simulink model "SLCI1_TP_Ericc3_Modele_Matlab_corrige_LMM"  (R2016b)
settings: Solver=ode3  StartTime=0.0  StopTime=5  FixedStep=0.01  RelTol=1e-3  EnableMultiTasking=on
settings Model: Creator=Mathieu  LastModifiedBy=emiliendurif
settings DataIOCC: LimitDataPoints=on  SaveFormat=Array
settings OptimizationCC: LifeSpan=inf
settings DebuggingCC: SFUnexpectedBacktrackingDiag=warning  SFNoUnconditionalDefaultTransitionDiag=warning  SFExecutionAtInitializationDiag=none
settings HardwareCC: ProdBitPerPointer=32  ProdBitPerSizeT=32  ProdBitPerPtrDiffT=32  ProdLargestAtomicFloat=None  ProdIntDivRoundTo=Undefined  ProdEndianess=Unspecified  ProdWordSize=32  ProdHWDeviceType=32-bit Generic
settings ModelReferenceCC: PropagateSignalLabelsOutOfModel=off
settings GRTTargetCC: TargetLangStandard=C89/C90 (ANSI)  GeneratePreprocessorConditionals=Disable all
settings ConfigComp: CovMetricSettings=dw  CovHtmlReporting=on  CovSaveCumulativeToWorkspaceVar=on  CovSaveSingleToWorkspaceVar=on  CovExternalEMLEnable=off

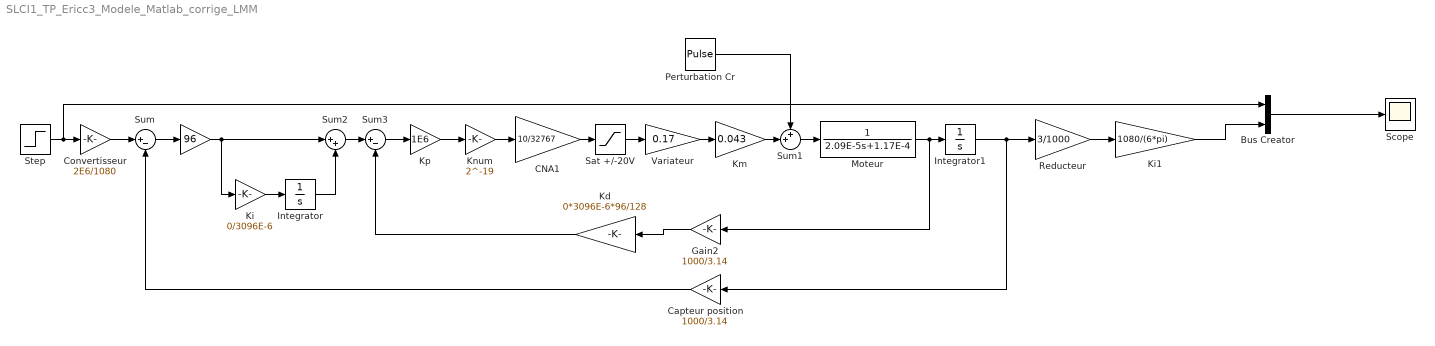
== system SLCI1_TP_Ericc3_Modele_Matlab_corrige_LMM ==
  " " : Gain  Gain=96
  Bus Creator : BusCreator  Inputs=2
  CNA1 : Gain  Gain=10/32767
  "Capteur position " : Gain  Gain=1000/3.14
  Convertisseur : Gain  Gain=2E6/1080
  Gain2 : Gain  Gain=1000/3.14
  Integrator : Integrator
  Integrator1 : Integrator
  Kd : Gain  Gain=0*3096E-6*96/128
  Ki : Gain  Gain=0/3096E-6
  Ki1 : Gain  Gain=1080/(6*pi)
  Km : Gain  Gain=0.043
  Knum : Gain  Gain=2^-19
  Kp : Gain  Gain=1E6
  Moteur : TransferFcn  Denominator=[2.09E-5 1.17E-4]
  "Perturbation Cr " : DiscretePulseGenerator  PulseType=Time based  Amplitude=0  Period=10
  Reducteur : Gain  Gain=3/1000
  Sat +/-20V : Saturate  UpperLimit=20  LowerLimit=-20
  Scope : Scope
  Step : Step  Time=0  After=30  SampleTime=0
  Sum : Sum  Inputs=|+-
  Sum1 : Sum  Inputs=++|
  Sum2 : Sum  Inputs=|++
  Sum3 : Sum  Inputs=|+-
  "Variateur " : Gain  Gain=0.17
  wires:
  Convertisseur/1 -> Sum/1
  Step/1 -> Bus Creator/1, Convertisseur/1
  "Variateur "/1 -> Km/1
  Km/1 -> Sum1/2
  Moteur/1 -> Integrator1/1, Gain2/1
  Integrator1/1 -> "Capteur position "/1, Reducteur/1
  Reducteur/1 -> Ki1/1
  Ki1/1 -> Bus Creator/2
  Bus Creator/1 -> Scope/1
  "Capteur position "/1 -> Sum/2
  "Perturbation Cr "/1 -> Sum1/1
  Sum/1 -> " "/1
  " "/1 -> Ki/1, Sum2/1
  Sum2/1 -> Sum3/1
  Integrator/1 -> Sum2/2
  Ki/1 -> Integrator/1
  Sum1/1 -> Moteur/1
  Knum/1 -> CNA1/1
  CNA1/1 -> Sat +/-20V/1
  Sat +/-20V/1 -> "Variateur "/1
  Gain2/1 -> Kd/1
  Kd/1 -> Sum3/2
  Sum3/1 -> Kp/1
  Kp/1 -> Knum/1
